simulink model "gain_sched_sim"  (R2021b)
settings: Solver=VariableStepAuto  StartTime=0.0  StopTime=3000  RelTol=1e-3
values from neighbouring files (symbols this model uses):
  params = struct    [run_gain_sched_popt.m]    (also in test_gain_sched_sim.m; test_run_simulation.m)
  Ts = 1    [gen_input_secs.m]    (also in run_gain_sched_popt.m = diff(t(1:2)); run_simulation.m = diff(t(1:2)); test_gain_sched_sim.m; test_run_simulation.m = diff(t(1:2)))
libraries: simulink x1
settings Model: Creator=billtubbs  LastModifiedBy=billtubbs

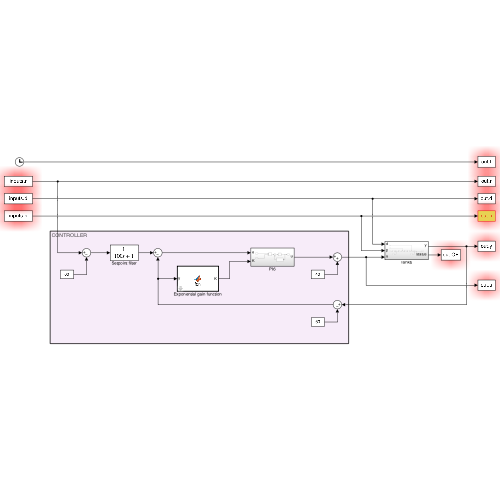
[thumbnail: Simulink's stored preview of the top-level diagram]
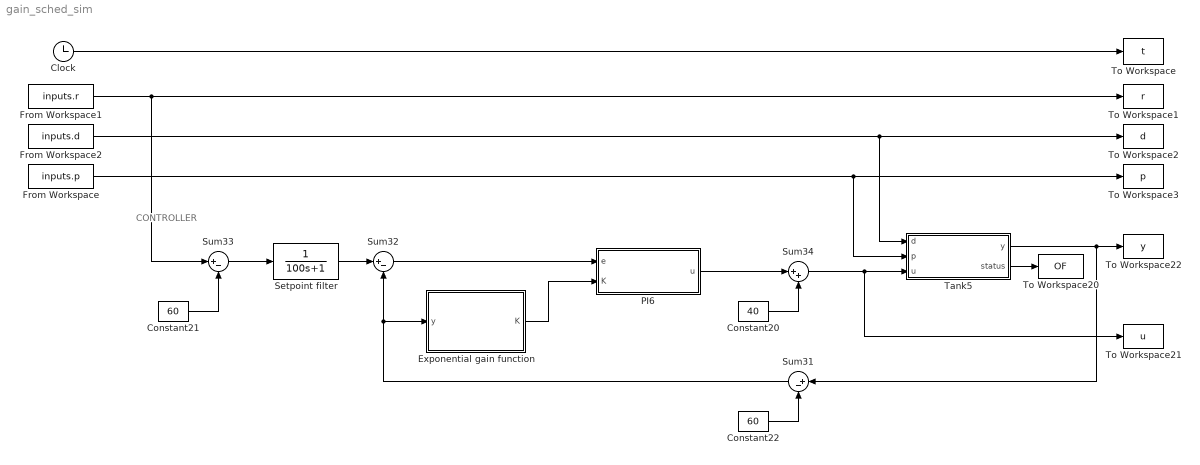
== system gain_sched_sim ==
  note: CONTROLLER
  Clock : Clock
  Constant20 : Constant  Value=40
  Constant21 : Constant  Value=60
  Constant22 : Constant  Value=60
  Exponential gain function : MATLAB Function  TreatAsAtomicUnit=on  mask{a=params.a, b=params.b, c=params.c}
  From Workspace : FromWorkspace  VariableName=inputs.p
  From Workspace1 : FromWorkspace  VariableName=inputs.r
  From Workspace2 : FromWorkspace  VariableName=inputs.d
  PI6 : Subsystem
  Setpoint filter : TransferFcn  Denominator=[100 1]
  Sum31 : Sum  Inputs=|+-
  Sum32 : Sum  Inputs=|+-
  Sum33 : Sum  Inputs=|+-
  Sum34 : Sum  Inputs=|++
  Tank5 : Subsystem
  To Workspace : ToWorkspace  VariableName=t  SampleTime=Ts
  To Workspace1 : ToWorkspace  VariableName=r  SampleTime=Ts
  To Workspace2 : ToWorkspace  VariableName=d  SampleTime=Ts
  To Workspace20 : ToWorkspace  VariableName=OF  SampleTime=Ts
  To Workspace21 : ToWorkspace  VariableName=u  SampleTime=Ts
  To Workspace22 : ToWorkspace  VariableName=y  SampleTime=Ts
  To Workspace3 : ToWorkspace  VariableName=p  SampleTime=Ts
  wires:
  PI6/1(u) -> Sum34/1
  Sum32/1 -> PI6/1(e)
  Tank5/2(status) -> To Workspace20/1
  From Workspace1/1 -> To Workspace1/1, Sum33/1
  Constant20/1 -> Sum34/2
  From Workspace/1 -> Tank5/2(p), To Workspace3/1
  Tank5/1(y) -> Sum31/1, To Workspace22/1
  Constant22/1 -> Sum31/2
  Sum34/1 -> Tank5/3(u), To Workspace21/1
  Sum31/1 -> Sum32/2, Exponential gain function/1(y)
  Sum33/1 -> Setpoint filter/1
  Constant21/1 -> Sum33/2
  From Workspace2/1 -> Tank5/1(d), To Workspace2/1
  Exponential gain function/1(K) -> PI6/2(K)
  Setpoint filter/1 -> Sum32/1
  Clock/1 -> To Workspace/1

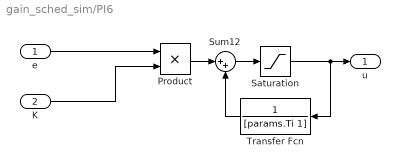
== system gain_sched_sim/PI6 ==
  e : Inport
  K : Inport  Port=2
  Product : Product
  Saturation : Saturate  UpperLimit=60  LowerLimit=-40
  Sum12 : Sum  Inputs=|++
  Transfer Fcn : TransferFcn  Numerator=1  Denominator=[params.Ti 1]
  u : Outport
  wires:
  e/1 -> Product/1
  Transfer Fcn/1 -> Sum12/2
  Product/1 -> Sum12/1
  Sum12/1 -> Saturation/1
  Saturation/1 -> Transfer Fcn/1, u/1
  K/1 -> Product/2

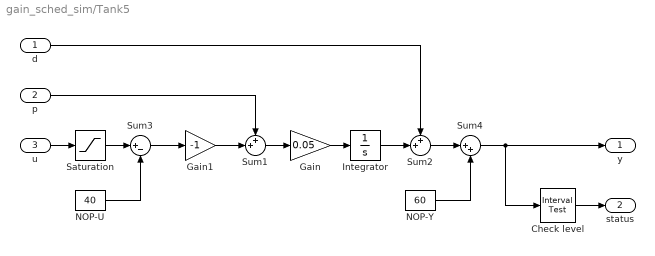
== system gain_sched_sim/Tank5 ==
  d : Inport
  p : Inport  Port=2
  u : Inport  Port=3
  Check level : simulink/Logic and Bit Operations/Interval Test  IntervalClosedRight=on  uplimit=100  IntervalClosedLeft=on  lowlimit=0  OutDataTypeStr=boolean
  Gain : Gain  Gain=0.05
  Gain1 : Gain  Gain=-1
  Integrator : Integrator
  NOP-U : Constant  Value=40
  NOP-Y : Constant  Value=60
  Saturation : Saturate  UpperLimit=100  LowerLimit=0
  Sum1 : Sum  Inputs=++|
  Sum2 : Sum  Inputs=++|
  Sum3 : Sum  Inputs=|+-
  Sum4 : Sum  Inputs=|++
  y : Outport
  status : Outport  Port=2
  wires:
  d/1 -> Sum2/1
  Gain/1 -> Integrator/1
  p/1 -> Sum1/1
  Integrator/1 -> Sum2/2
  Sum2/1 -> Sum4/1
  u/1 -> Saturation/1
  Sum1/1 -> Gain/1
  NOP-U/1 -> Sum3/2
  NOP-Y/1 -> Sum4/2
  Sum4/1 -> y/1, Check level/1
  Check level/1 -> status/1
  Saturation/1 -> Sum3/1
  Gain1/1 -> Sum1/2
  Sum3/1 -> Gain1/1

== matlab function gain_sched_sim/Exponential gain function ==
  data: y input; K output; a parameter; b parameter; c parameter
function K = fcn(y, a, b, c)
% Exponential function for gain scheduling of the form
%
%   K = a + b .* (exp(-y ./ c) + exp((y - y_max) ./ c));
%
% Where a, b, and c are constants.
%
% For example. To achieve the following requirements:
% At y = 0, gain = -5
% At y = 50, gain = -0.1
% At y = 100, gain = -5
%
% Set:
%  a = -0.1;
%  b = -4.9;
%  c = 5;
%
% Note: normal operating point, which is 60, must
%   be added to y in this formula.
%

    K = a + b .* (exp(-(y + 60) ./ c) + exp((y - 40) ./ c));

end
